simulink model "Nonlinear_Stabilization"  (R2020b)
settings: Solver=VariableStepAuto  StartTime=0.0  StopTime=400  RelTol=1e-3
settings Model: Creator=zhiyao  LastModifiedBy=zhiyao

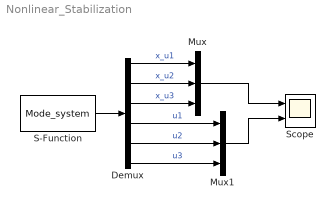
== system Nonlinear_Stabilization ==
  Demux : Demux  Outputs=6
  Mux : Mux  Inputs=3
  Mux1 : Mux  Inputs=3
  S-Function : S-Function  FunctionName=Mode_system  SFunctionDeploymentMode=off  EnableBusSupport=off
  Scope : Scope  NumInputPorts=2
  wires:
  S-Function/1 -> Demux/1
  Demux/1 -> Mux/1  "x_u1"
  Demux/2 -> Mux/2  "x_u2"
  Demux/3 -> Mux/3  "x_u3"
  Demux/4 -> Mux1/1  "u1"
  Demux/5 -> Mux1/2  "u2"
  Demux/6 -> Mux1/3  "u3"
  Mux/1 -> Scope/1
  Mux1/1 -> Scope/2
